simulink model "sampleModel1844"  (R2023a)
settings: Solver=VariableStepAuto  StartTime=0.0  StopTime=10.0  RelTol=1e-3
libraries: hdlsllib x12, simulink x3
settings Model: Creator=user1  LastModifiedBy=user1

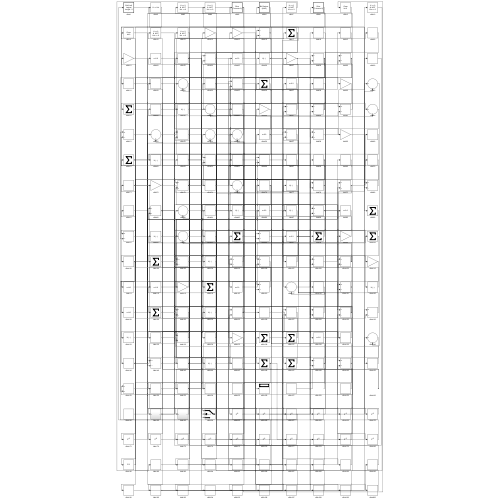
[thumbnail: Simulink's stored preview of the top-level diagram]
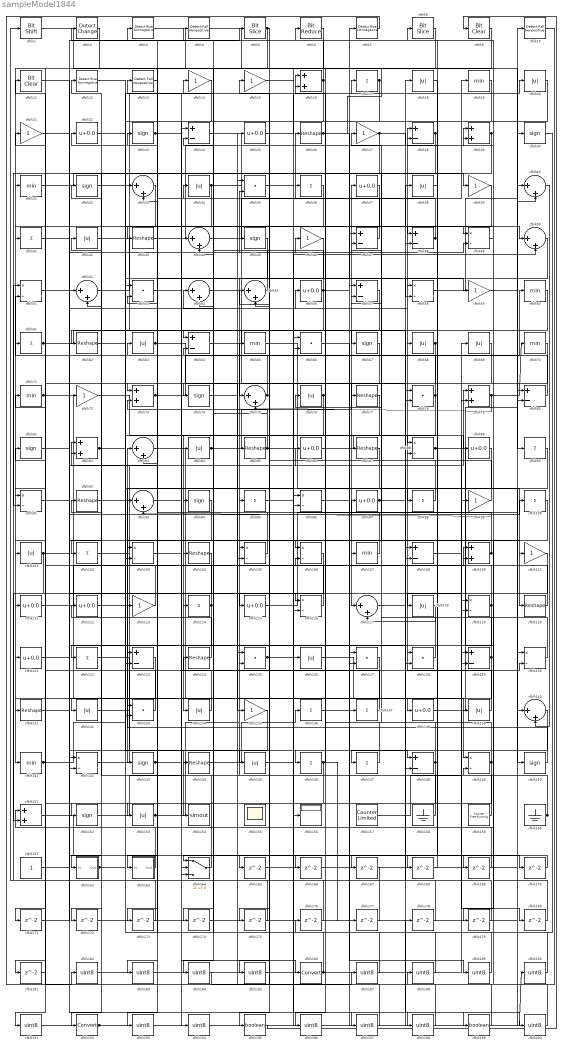
== system sampleModel1844 ==
  cfblk1 : hdlsllib/Logic and Bit Operations/Bit Shift  mode=Shift Left Logical  N=0
  cfblk10 : hdlsllib/Logic and Bit Operations/Detect Fall Nonpositive  vinit=0  OutDataTypeStr=boolean
  cfblk{17,36,41,61,90,95,98,100,102,114,122,136..137,146..147} (15 alike) : Sum  Inputs=+
  cfblk{18,20,34,38,42,63,68..69,76,84,101,118,126,132,134,139,145,153} (18 alike) : Abs  SaturateOnIntegerOverflow=off
  cfblk{49,51,58,88,91,96,103,105..106,116,119,130,142,149} (14 alike) : Product  Inputs=*/  RndMeth=Zero  SaturateOnIntegerOverflow=on
  cfblk{26,43,62,77,85,87,92,104,120,124,131,144} (12 alike) : Reshape
  cfblk{19,31,60,65,70..71,107,141} (8 alike) : MinMax
  cfblk{24,28,47..48,57,64,80,108,123,129,148} (11 alike) : Sum  Inputs=+-
  cfblk{16,29,73,79,82,109,151} (7 alike) : Sum
  cfblk11 : simulink/Logic and Bit Operations/Bit Clear  iBit=0
      settings: LibrarySourceBlock=|
      | hdlsllib/Logic and Bit
      | Operations/Bit Clear
  cfblk{14..15,21,27,39,46,59,72,99,110,113,135} (12 alike) : Gain
  cfblk{22,25,37,56,86,89,97,111..112,115,121,138} (12 alike) : Bias  Bias=0.0  SaturateOnIntegerOverflow=off
  cfblk{33,40,44,50,52,54..55,75,83,93,117,140} (12 alike) : Sum  Inputs=|++
  cfblk12 : hdlsllib/Logic and Bit Operations/Detect Rise Nonnegative  vinit=0  OutDataTypeStr=boolean
  cfblk{35,53,66,78,125,127..128,133} (8 alike) : DotProduct  OutDataTypeStr=Inherit: Inherit via internal rule
  cfblk13 : hdlsllib/Logic and Bit Operations/Detect Fall Nonpositive  vinit=0  OutDataTypeStr=boolean
  cfblk{23,30,32,45,67,74,81,94,143,150,152} (11 alike) : Signum
  cfblk154 : ToWorkspace  VariableName=simout  SaveFormat=Timeseries  SampleTime=-1
  cfblk155 : Scope
      settings: Floating=on
  cfblk156 : Display
  cfblk157 : hdlsllib/Sources/Counter Limited  uplimit=7  tsamp=-1
  cfblk158 : Ground
  cfblk159 : hdlsllib/Sources/Counter Free-Running  NumBits=16  tsamp=-1
  cfblk160 : Ground
  cfblk161 : Constant  SampleTime=-1
  cfblk162 : Subsystem
      settings: LibrarySourceBlock=|
      | hdlsllib/Ports &
      | Subsystems/Subsystem
  cfblk163 : Subsystem
      settings: LibrarySourceBlock=|
      | hdlsllib/Ports &
      | Subsystems/Subsystem
  cfblk164 : Switch  SaturateOnIntegerOverflow=off  InputSameDT=off
  cfblk{165..181} (17 alike) : Delay  SampleTime=1
  cfblk{182..185,187..191,193..194,196..198,200} (15 alike) : DataTypeConversion  OutDataTypeStr=uint8  SaturateOnIntegerOverflow=off  RndMeth=Floor
  cfblk186 : DataTypeConversion  SaturateOnIntegerOverflow=off  RndMeth=Floor
  cfblk192 : DataTypeConversion  SaturateOnIntegerOverflow=off  RndMeth=Floor
  cfblk195 : DataTypeConversion  OutDataTypeStr=boolean  SaturateOnIntegerOverflow=off  RndMeth=Floor
  cfblk199 : DataTypeConversion  OutDataTypeStr=boolean  SaturateOnIntegerOverflow=off  RndMeth=Floor
  cfblk2 : simulink/Logic and Bit Operations/Detect Change  vinit=0  OutDataTypeStr=boolean
      settings: LibrarySourceBlock=|
      | hdlsllib/Logic and Bit
      | Operations/Detect
      | Change
  cfblk3 : hdlsllib/Logic and Bit Operations/Detect Rise Nonnegative  vinit=0  OutDataTypeStr=boolean
  cfblk4 : hdlsllib/Logic and Bit Operations/Detect Fall Nonpositive  vinit=0  OutDataTypeStr=boolean
  cfblk5 : hdlsllib/Logic and Bit Operations/Bit Slice  lidx=7  ridx=0
  cfblk6 : hdlsllib/Logic and Bit Operations/Bit Reduce  mode=AND
  cfblk7 : hdlsllib/Logic and Bit Operations/Detect Rise Nonnegative  vinit=0  OutDataTypeStr=boolean
  cfblk8 : hdlsllib/Logic and Bit Operations/Bit Slice  lidx=7  ridx=0
  cfblk9 : simulink/Logic and Bit Operations/Bit Clear  iBit=0
      settings: LibrarySourceBlock=|
      | hdlsllib/Logic and Bit
      | Operations/Bit Clear
  wires:
  cfblk139/1 -> cfblk28/1
  cfblk61/1 -> cfblk64/1, cfblk105/2
  cfblk57/1 -> cfblk132/1
  cfblk124/1 -> cfblk52/2
  cfblk63/1 -> cfblk17/1, cfblk135/1
  cfblk144/1 -> cfblk136/1
  cfblk153/1 -> cfblk27/1, cfblk125/2
  cfblk73/1 -> cfblk60/1, cfblk45/1
  cfblk31/1 -> cfblk39/1
  cfblk145/1 -> cfblk126/1
  cfblk52/1 -> cfblk14/1
  cfblk88/1 -> cfblk151/1, cfblk180/1
  cfblk26/1 -> cfblk141/1, cfblk58/2
  cfblk47/1 -> cfblk26/1
  cfblk119/1 -> cfblk83/1, cfblk133/2
  cfblk76/1 -> cfblk83/2, cfblk106/1
  cfblk141/1 -> cfblk33/1, cfblk5/1
  cfblk163/1(Out1) -> cfblk81/1
  cfblk77/1 -> cfblk134/1
  cfblk19/1 -> cfblk48/1
  cfblk92/1 -> cfblk79/1
  cfblk146/1 -> cfblk16/1, cfblk152/1, cfblk177/1
  cfblk50/1 -> cfblk75/1
  cfblk71/1 -> cfblk138/1, cfblk128/2
  cfblk84/1 -> cfblk37/1, cfblk88/1
  cfblk79/1 -> cfblk70/1, cfblk75/2
  cfblk21/1 -> cfblk142/1
  cfblk142/1 -> cfblk69/1
  cfblk49/1 -> cfblk6/1
  cfblk58/1 -> cfblk30/1
  cfblk129/1 -> cfblk123/1, cfblk76/1, cfblk122/1, cfblk172/1
  cfblk134/1 -> cfblk71/1
  cfblk107/1 -> cfblk82/1
  cfblk159/1 -> cfblk85/1
  cfblk115/1 -> cfblk10/1
  cfblk5/1 -> cfblk174/1, cfblk175/1
  cfblk105/1 -> cfblk22/1
  cfblk90/1 -> cfblk143/1
  cfblk97/1 -> cfblk38/1, cfblk169/1, cfblk199/1
  cfblk133/1 -> cfblk12/1
  cfblk137/1 -> cfblk23/1
  cfblk138/1 -> cfblk40/2
  cfblk54/1 -> cfblk117/1
  cfblk104/1 -> cfblk151/2
  cfblk83/1 -> cfblk156/1
  cfblk25/1 -> cfblk20/1
  cfblk127/1 -> cfblk192/1
  cfblk120/1 -> cfblk109/1
  cfblk29/1 -> cfblk107/1, cfblk101/1
  cfblk64/1 -> cfblk67/1
  cfblk33/1 -> cfblk102/1
  cfblk152/1 -> cfblk24/1
  cfblk27/1 -> cfblk115/1, cfblk50/1
  cfblk6/1 -> cfblk31/1
  cfblk85/1 -> cfblk120/1, cfblk73/2, cfblk64/2
  cfblk102/1 -> cfblk97/1
  cfblk112/1 -> cfblk57/1
  cfblk60/1 -> cfblk162/1(In1)
  cfblk22/1 -> cfblk145/1
  cfblk122/1 -> cfblk154/1
  cfblk81/1 -> cfblk56/1
  cfblk111/1 -> cfblk47/1
  cfblk34/1 -> cfblk78/2, cfblk111/1
  cfblk24/1 -> cfblk137/1
  cfblk114/1 -> cfblk92/1, cfblk183/1
  cfblk91/1 -> cfblk116/1
  cfblk78/1 -> cfblk51/2, cfblk103/2
  cfblk40/1 -> cfblk140/2
  cfblk17/1 -> cfblk144/1, cfblk123/2
  cfblk32/1 -> cfblk49/1
  cfblk164/1 -> cfblk63/1
  cfblk20/1 -> cfblk94/1
  cfblk43/1 -> cfblk18/1
  cfblk8/1 -> cfblk33/2
  cfblk101/1 -> cfblk49/2, cfblk121/1, cfblk88/2
  cfblk18/1 -> cfblk98/1
  cfblk45/1 -> cfblk74/1
  cfblk113/1 -> cfblk21/1
  cfblk131/1 -> cfblk100/1
  cfblk125/1 -> cfblk15/1, cfblk50/2
  cfblk94/1 -> cfblk153/1
  cfblk93/1 -> cfblk46/1
  cfblk96/1 -> cfblk110/1
  cfblk46/1 -> cfblk163/1(In1)
  cfblk143/1 -> cfblk44/1, cfblk130/2
  cfblk53/1 -> cfblk186/1
  cfblk2/1 -> cfblk41/1
  cfblk39/1 -> cfblk131/1
  cfblk118/1 -> cfblk117/2
  cfblk150/1 -> cfblk93/1
  cfblk110/1 -> cfblk118/1
  cfblk62/1 -> cfblk16/2
  cfblk151/1 -> cfblk164/2
  cfblk56/1 -> cfblk13/1, cfblk29/1, cfblk104/1
  cfblk160/1 -> cfblk8/1, cfblk112/1
  cfblk15/1 -> cfblk148/1
  cfblk42/1 -> cfblk148/2
  cfblk12/1 -> cfblk59/1
  cfblk162/1(Out1) -> cfblk109/2, cfblk58/1
  cfblk82/1 -> cfblk96/2, cfblk108/2
  cfblk147/1 -> cfblk36/1
  cfblk86/1 -> cfblk89/1
  cfblk116/1 -> cfblk105/1
  cfblk89/1 -> cfblk114/1
  cfblk37/1 -> cfblk54/2
  cfblk132/1 -> cfblk146/1
  cfblk149/1 -> cfblk106/2, cfblk185/1
  cfblk74/1 -> cfblk68/1
  cfblk55/1 -> cfblk35/2
  cfblk109/1 -> cfblk82/2, cfblk103/1, cfblk93/2
  cfblk68/1 -> cfblk84/1, cfblk91/1
  cfblk99/1 -> cfblk57/2
  cfblk108/1 -> cfblk99/1
  cfblk130/1 -> cfblk34/1
  cfblk23/1 -> cfblk119/2, cfblk167/1
  cfblk4/1 -> cfblk116/2
  cfblk126/1 -> cfblk149/1
  cfblk148/1 -> cfblk77/1, cfblk128/1, cfblk191/1
  cfblk157/1 -> cfblk79/2
  cfblk3/1 -> cfblk80/1
  cfblk51/1 -> cfblk139/1
  cfblk98/1 -> cfblk55/1
  cfblk128/1 -> cfblk65/1
  cfblk140/1 -> cfblk147/1
  cfblk44/1 -> cfblk19/1
  cfblk117/1 -> cfblk108/1
  cfblk135/1 -> cfblk142/2
  cfblk28/1 -> cfblk62/1, cfblk73/1, cfblk91/2
  cfblk48/1 -> cfblk43/1, cfblk3/1
  cfblk70/1 -> cfblk133/1
  cfblk72/1 -> cfblk129/1
  cfblk16/1 -> cfblk113/1, cfblk2/1
  cfblk75/1 -> cfblk4/1, cfblk42/1
  cfblk158/1 -> cfblk32/1
  cfblk1/1 -> cfblk90/1
  cfblk59/1 -> cfblk80/2
  cfblk65/1 -> cfblk150/1
  cfblk161/1 -> cfblk86/1
  cfblk14/1 -> cfblk164/3
  cfblk121/1 -> cfblk72/1
  cfblk80/1 -> cfblk47/2
  cfblk69/1 -> cfblk165/1
  cfblk165/1 -> cfblk40/1
  cfblk41/1 -> cfblk166/1
  cfblk166/1 -> cfblk48/2
  cfblk167/1 -> cfblk1/1
  cfblk38/1 -> cfblk168/1
  cfblk168/1 -> cfblk28/2
  cfblk169/1 -> cfblk119/1
  cfblk136/1 -> cfblk170/1
  cfblk170/1 -> cfblk164/1
  cfblk123/1 -> cfblk171/1
  cfblk171/1 -> cfblk52/1
  cfblk172/1 -> cfblk96/1
  cfblk106/1 -> cfblk173/1
  cfblk173/1 -> cfblk51/1
  cfblk174/1 -> cfblk140/1
  cfblk175/1 -> cfblk44/2
  cfblk30/1 -> cfblk176/1
  cfblk176/1 -> cfblk24/2
  cfblk177/1 -> cfblk55/2
  cfblk178/1 -> cfblk78/1
  cfblk100/1 -> cfblk179/1
  cfblk179/1 -> cfblk35/1
  cfblk180/1 -> cfblk29/2
  cfblk67/1 -> cfblk181/1
  cfblk181/1 -> cfblk61/1
  cfblk7/1 -> cfblk182/1
  cfblk182/1 -> cfblk25/1
  cfblk183/1 -> cfblk7/1
  cfblk87/1 -> cfblk184/1
  cfblk185/1 -> cfblk87/1
  cfblk186/1 -> cfblk129/2, cfblk124/1
  cfblk184/1 -> cfblk187/1
  cfblk187/1 -> cfblk53/1
  cfblk10/1 -> cfblk188/1
  cfblk188/1 -> cfblk53/2
  cfblk66/1 -> cfblk189/1
  cfblk189/1 -> cfblk54/1
  cfblk190/1 -> cfblk66/1
  cfblk191/1 -> cfblk66/2
  cfblk192/1 -> cfblk190/1, cfblk178/1
  cfblk13/1 -> cfblk193/1
  cfblk193/1 -> cfblk127/1
  cfblk103/1 -> cfblk194/1
  cfblk194/1 -> cfblk127/2
  cfblk36/1 -> cfblk195/1
  cfblk195/1 -> cfblk9/1
  cfblk9/1 -> cfblk196/1
  cfblk196/1 -> cfblk130/1
  cfblk95/1 -> cfblk197/1
  cfblk197/1 -> cfblk125/1
  cfblk35/1 -> cfblk198/1
  cfblk198/1 -> cfblk95/1
  cfblk199/1 -> cfblk11/1
  cfblk11/1 -> cfblk200/1
  cfblk200/1 -> cfblk149/2

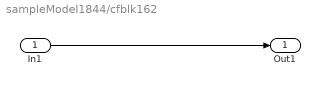
== system sampleModel1844/cfblk162 ==
  In1 : Inport
  Out1 : Outport
  wires:
  In1/1 -> Out1/1

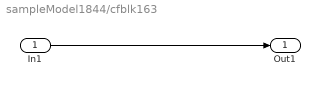
== system sampleModel1844/cfblk163 ==
  In1 : Inport
  Out1 : Outport
  wires:
  In1/1 -> Out1/1
